simulink model "PF70mmDuctFanP"  (R2018b)
settings: Solver=ode4  StartTime=0.0  StopTime=10.0  RelTol=1e-3
libraries: simulink x1, vrlib x1
settings Model: Creator=sweat  LastModifiedBy=39926

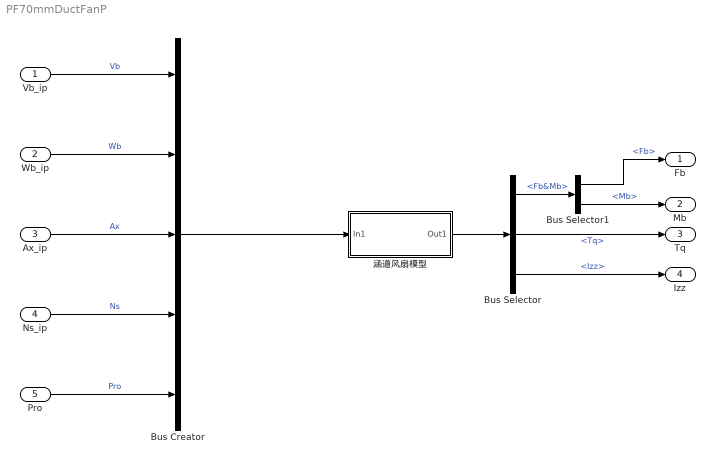
== system PF70mmDuctFanP ==
  Vb_ip : Inport  PortDimensions=3
  Wb_ip : Inport  Port=2  PortDimensions=3
  Ax_ip : Inport  Port=3  PortDimensions=3
  Ns_ip : Inport  Port=4  PortDimensions=1
  Pro : Inport  Port=5  PortDimensions=1
  Bus Selector : BusSelector  OutputSignals=Fb&Mb,Tq,Izz
  Bus Selector1 : BusSelector  OutputSignals=Fb,Mb
  Bus Creator : BusCreator  Inputs=5
  "涵道风扇模型 " : Subsystem  mask{Fratio=1.125, Mratio=0.975, Tqratio=0.4, Izz=0.00000309}
      mask prompts: Fratio "涵道风扇气动力修正系数"; Mratio "涵道风扇气动力矩修正系数"; Tqratio "涵道风扇扭矩修正系数"; Izz "涵道风扇转动惯量"
  Fb : Outport
  Mb : Outport  Port=2
  Tq : Outport  Port=3
  Izz : Outport  Port=4
  wires:
  Vb_ip/1 -> Bus Creator/1  "Vb"
  Wb_ip/1 -> Bus Creator/2  "Wb"
  Ax_ip/1 -> Bus Creator/3  "Ax"
  Ns_ip/1 -> Bus Creator/4  "Ns"
  Pro/1 -> Bus Creator/5  "Pro"
  Bus Creator/1 -> "涵道风扇模型 "/1(In1)
  "涵道风扇模型 "/1(Out1) -> Bus Selector/1
  Bus Selector/1 -> Bus Selector1/1  "<Fb&Mb>"
  Bus Selector1/1 -> Fb/1  "<Fb>"
  Bus Selector1/2 -> Mb/1  "<Mb>"
  Bus Selector/2 -> Tq/1  "<Tq>"
  Bus Selector/3 -> Izz/1  "<Izz>"

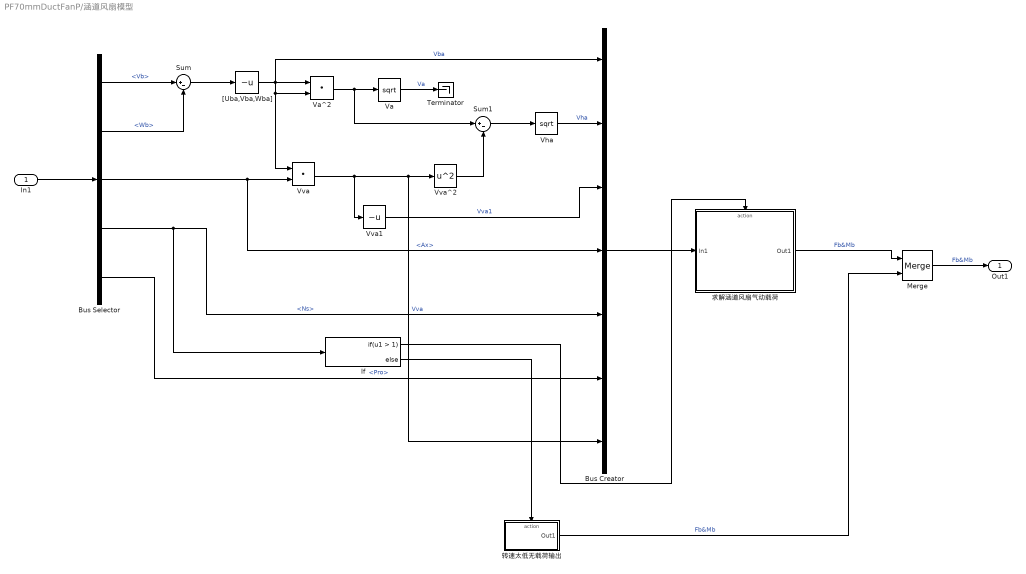
== system PF70mmDuctFanP/涵道风扇模型  ==
  In1 : Inport
  Bus Creator : BusCreator  Inputs=7
  Bus Selector : BusSelector  OutputSignals=Vb,Wb,Ax,Ns,Pro
  If : If  IfExpression=u1 > 1
  Merge : Merge
  Sum : Sum  Inputs=|+-
  Sum1 : Sum  Inputs=|+-
  Terminator : Terminator
  Va : Sqrt  SaturateOnIntegerOverflow=on
  Va^2 : DotProduct  InputSameDT=on  OutDataTypeStr=Inherit: Inherit via internal rule
  Vha : Sqrt  SaturateOnIntegerOverflow=on
  Vva : DotProduct  InputSameDT=on  OutDataTypeStr=Inherit: Inherit via internal rule
  Vva1 : UnaryMinus
  Vva^2 : Math  Operator=square  SaturateOnIntegerOverflow=on
  "[Uba,Vba,Wba]" : UnaryMinus
  求解涵道风扇气动载荷 : Subsystem  TreatAsAtomicUnit=on
  转速太低无载荷输出 : Subsystem  TreatAsAtomicUnit=on
  Out1 : Outport
  wires:
  Bus Selector/1 -> Sum/1  "<Vb>"
  In1/1 -> Bus Selector/1
  Bus Selector/2 -> Sum/2  "<Wb>"
  Sum/1 -> "[Uba,Vba,Wba]"/1
  "[Uba,Vba,Wba]"/1 -> Bus Creator/1, Vva/1, Va^2/2, Va^2/1  "Vba"
  Bus Selector/3 -> Bus Creator/4, Vva/2  "<Ax>"
  Va^2/1 -> Sum1/1, Va/1
  Vva/1 -> Bus Creator/7, Vva^2/1, Vva1/1  "Vva"
  Vva^2/1 -> Sum1/2
  Sum1/1 -> Vha/1
  Vha/1 -> Bus Creator/2  "Vha"
  Vva1/1 -> Bus Creator/3  "Vva1"
  Bus Selector/4 -> Bus Creator/5, If/1  "<Ns>"
  If/1 -> 求解涵道风扇气动载荷/Action
  If/2 -> 转速太低无载荷输出/Action
  Bus Selector/5 -> Bus Creator/6  "<Pro>"
  Bus Creator/1 -> 求解涵道风扇气动载荷/1(In1)
  求解涵道风扇气动载荷/1(Out1) -> Merge/1  "Fb&Mb"
  转速太低无载荷输出/1(Out1) -> Merge/2  "Fb&Mb"
  Va/1 -> Terminator/1  "Va"
  Merge/1 -> Out1/1  "Fb&Mb"

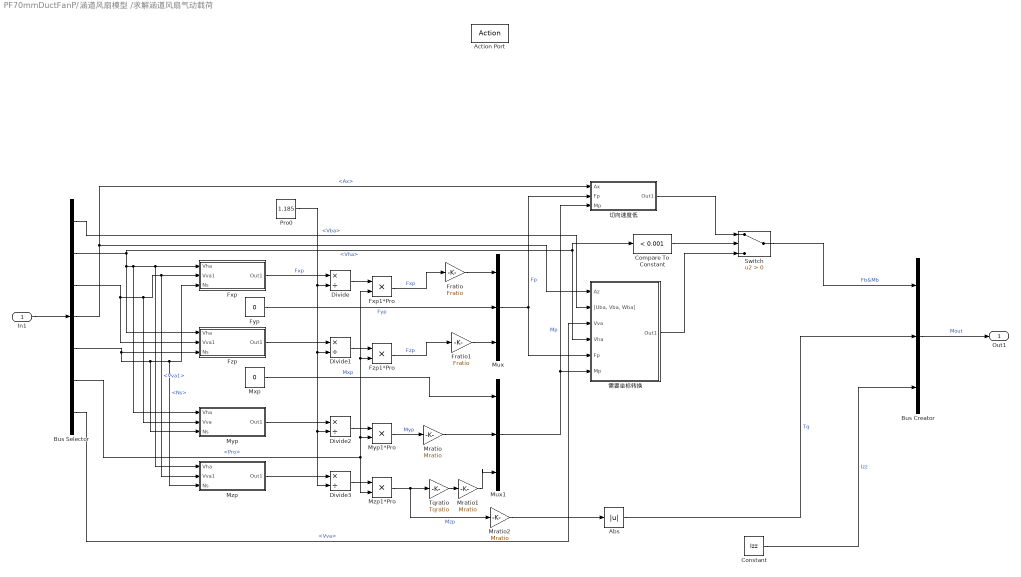
== system PF70mmDuctFanP/涵道风扇模型 /求解涵道风扇气动载荷 ==
  In1 : Inport
  Action Port : ActionPort  ActionType=then
  Abs : Abs
  Bus Creator : BusCreator  Inputs=3
  Bus Selector : BusSelector  OutputSignals=Vba,Vha,Vva1,Ax,Ns,Pro,Vva
  Compare To Constant : simulink/Logic and Bit Operations/Compare To Constant  relop=<  const=0.001  OutDataTypeStr=boolean
  Constant : Constant  Value=Izz
  Divide{,1..3} (4 alike) : Product  Inputs=*/
  Fratio : Gain  Gain=Fratio
  Fratio1 : Gain  Gain=Fratio
  Fxp : Subsystem
  Fxp1*Pro : Product
  Fyp : Constant  Value=0
  Fzp : Subsystem
  Fzp1*Pro : Product
  Mratio : Gain  Gain=Mratio
  Mratio1 : Gain  Gain=Mratio
  Mratio2 : Gain  Gain=Mratio
  Mux : Mux  Inputs=3
  Mux1 : Mux  Inputs=3
  Mxp : Constant  Value=0
  Myp : Subsystem
  Myp1*Pro : Product
  Mzp : Subsystem
  Mzp1*Pro : Product
  Pro0 : Constant  Value=1.185
  Switch : Switch  Criteria=u2 > Threshold
  Tqratio : Gain  Gain=Tqratio
  切向速度低 : Subsystem
  需要坐标转换 : Subsystem
  Out1 : Outport
  wires:
  In1/1 -> Bus Selector/1
  Bus Selector/2 -> Fzp/1(Vha), Myp/1(Vha), Mzp/1(Vha), Fxp/1(Vha), 需要坐标转换/4(Vha), Compare To Constant/1  "<Vha>"
  Bus Selector/3 -> Myp/2(Vva), Mzp/2(Vva1), Fxp/2(Vva1), Fzp/2(Vva1)  "<Vva1>"
  Bus Selector/5 -> Fzp/3(Ns), Myp/3(Ns), Mzp/3(Ns), Fxp/3(Ns)  "<Ns>"
  Fyp/1 -> Mux/2  "Fyp"
  Fxp/1(Out1) -> Divide/1  "Fxp"
  Fzp/1(Out1) -> Divide1/1
  Myp/1(Out1) -> Divide2/1
  Mzp/1(Out1) -> Divide3/1
  Pro0/1 -> Divide3/2, Divide2/2, Divide1/2, Divide/2
  Divide/1 -> Fxp1*Pro/1
  Fxp1*Pro/1 -> Fratio/1  "Fxp"
  Divide1/1 -> Fzp1*Pro/1
  Fzp1*Pro/1 -> Fratio1/1  "Fzp"
  Bus Selector/6 -> Mzp1*Pro/2, Myp1*Pro/2, Fzp1*Pro/2, Fxp1*Pro/2  "<Pro>"
  Divide2/1 -> Myp1*Pro/1
  Myp1*Pro/1 -> Mratio/1  "Myp"
  Divide3/1 -> Mzp1*Pro/1
  Bus Selector/4 -> 需要坐标转换/1(Az), 切向速度低/1(Ax)  "<Ax>"
  Mux/1 -> 需要坐标转换/5(Fp), 切向速度低/2(Fp)  "Fp"
  Mux1/1 -> 需要坐标转换/6(Mp), 切向速度低/3(Mp)  "Mp"
  Bus Selector/1 -> 需要坐标转换/2("[Uba, Vba, Wba]")  "<Vba>"
  Bus Selector/7 -> 需要坐标转换/3(Vva)  "<Vva>"
  Compare To Constant/1 -> Switch/2
  需要坐标转换/1(Out1) -> Switch/3
  Abs/1 -> Bus Creator/2  "Tq"
  Mzp1*Pro/1 -> Mratio2/1, Tqratio/1  "Mzp"
  Fratio/1 -> Mux/1
  Fratio1/1 -> Mux/3
  Tqratio/1 -> Mratio1/1
  Mratio/1 -> Mux1/2
  Mratio1/1 -> Mux1/3
  Mratio2/1 -> Abs/1
  Constant/1 -> Bus Creator/3  "Izz"
  Switch/1 -> Bus Creator/1  "Fb&Mb"
  Bus Creator/1 -> Out1/1  "Mout"
  切向速度低/1(Out1) -> Switch/1
  Mxp/1 -> Mux1/1  "Mxp"

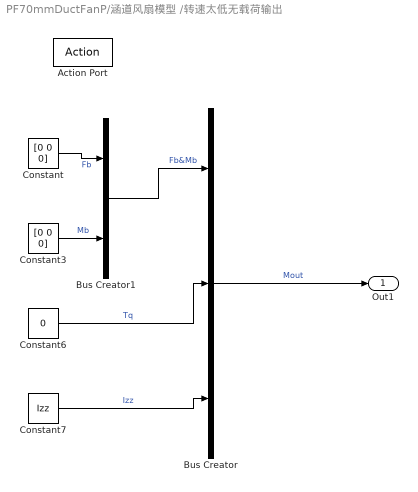
== system PF70mmDuctFanP/涵道风扇模型 /转速太低无载荷输出 ==
  Action Port : ActionPort  ActionType=else
  Bus Creator : BusCreator  Inputs=3
  Bus Creator1 : BusCreator  Inputs=2
  Constant : Constant  Value=[0 0 0]
  Constant3 : Constant  Value=[0 0 0]
  Constant6 : Constant  Value=0
  Constant7 : Constant  Value=Izz
  Out1 : Outport
  wires:
  Constant6/1 -> Bus Creator/2  "Tq"
  Constant7/1 -> Bus Creator/3  "Izz"
  Bus Creator/1 -> Out1/1  "Mout"
  Constant/1 -> Bus Creator1/1  "Fb"
  Constant3/1 -> Bus Creator1/2  "Mb"
  Bus Creator1/1 -> Bus Creator/1  "Fb&Mb"

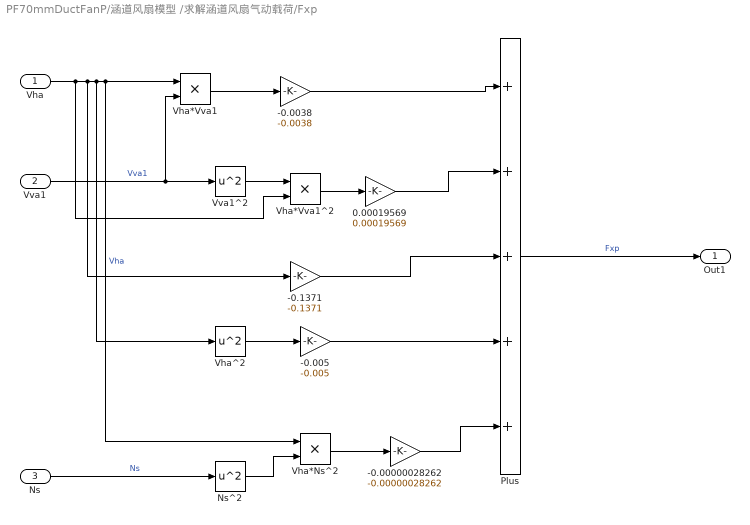
== system PF70mmDuctFanP/涵道风扇模型 /求解涵道风扇气动载荷/Fxp ==
  Vha : Inport
  Vva1 : Inport  Port=2
  Ns : Inport  Port=3
  -0.00000028262 : Gain  Gain=-0.00000028262
  -0.0038 : Gain  Gain=-0.0038
  -0.005 : Gain  Gain=-0.005
  -0.1371 : Gain  Gain=-0.1371
  0.00019569 : Gain  Gain=0.00019569
  Ns^2 : Math  Operator=square  SaturateOnIntegerOverflow=on
  Plus : Sum  Inputs=+++++
  Vha*Ns^2 : Product
  Vha*Vva1 : Product
  Vha*Vva1^2 : Product
  Vha^2 : Math  Operator=square  SaturateOnIntegerOverflow=on
  Vva1^2 : Math  Operator=square  SaturateOnIntegerOverflow=on
  Out1 : Outport
  wires:
  Vha/1 -> Vha*Vva1^2/2, -0.1371/1, Vha^2/1, Vha*Ns^2/1, Vha*Vva1/1  "Vha"
  Vva1/1 -> Vva1^2/1, Vha*Vva1/2  "Vva1"
  Vha*Vva1/1 -> -0.0038/1
  -0.0038/1 -> Plus/1
  Ns/1 -> Ns^2/1  "Ns"
  Vva1^2/1 -> Vha*Vva1^2/1
  Vha*Vva1^2/1 -> 0.00019569/1
  0.00019569/1 -> Plus/2
  -0.1371/1 -> Plus/3
  Vha^2/1 -> -0.005/1
  -0.005/1 -> Plus/4
  Ns^2/1 -> Vha*Ns^2/2
  Vha*Ns^2/1 -> -0.00000028262/1
  -0.00000028262/1 -> Plus/5
  Plus/1 -> Out1/1  "Fxp"

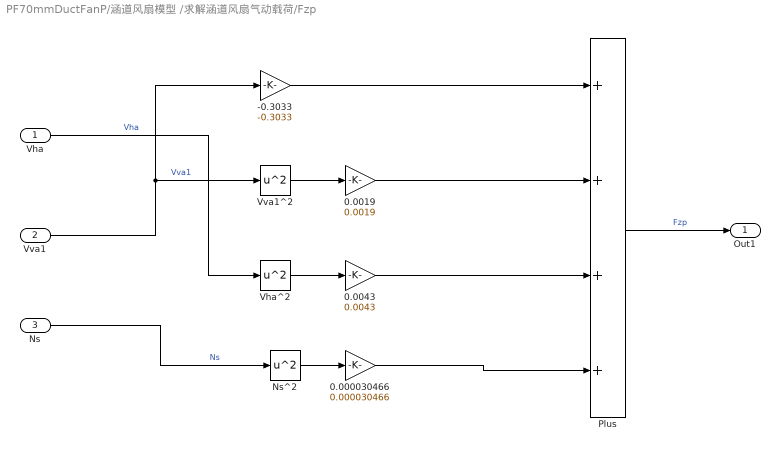
== system PF70mmDuctFanP/涵道风扇模型 /求解涵道风扇气动载荷/Fzp ==
  Vha : Inport
  Vva1 : Inport  Port=2
  Ns : Inport  Port=3
  -0.3033 : Gain  Gain=-0.3033
  0.000030466 : Gain  Gain=0.000030466
  0.0019 : Gain  Gain=0.0019
  0.0043 : Gain  Gain=0.0043
  Ns^2 : Math  Operator=square  SaturateOnIntegerOverflow=on
  Plus : Sum  Inputs=++++
  Vha^2 : Math  Operator=square  SaturateOnIntegerOverflow=on
  Vva1^2 : Math  Operator=square  SaturateOnIntegerOverflow=on
  Out1 : Outport
  wires:
  Vha/1 -> Vha^2/1  "Vha"
  Vva1/1 -> -0.3033/1, Vva1^2/1  "Vva1"
  Ns/1 -> Ns^2/1  "Ns"
  -0.3033/1 -> Plus/1
  Vva1^2/1 -> 0.0019/1
  0.0019/1 -> Plus/2
  Vha^2/1 -> 0.0043/1
  0.0043/1 -> Plus/3
  Ns^2/1 -> 0.000030466/1
  0.000030466/1 -> Plus/4
  Plus/1 -> Out1/1  "Fzp"

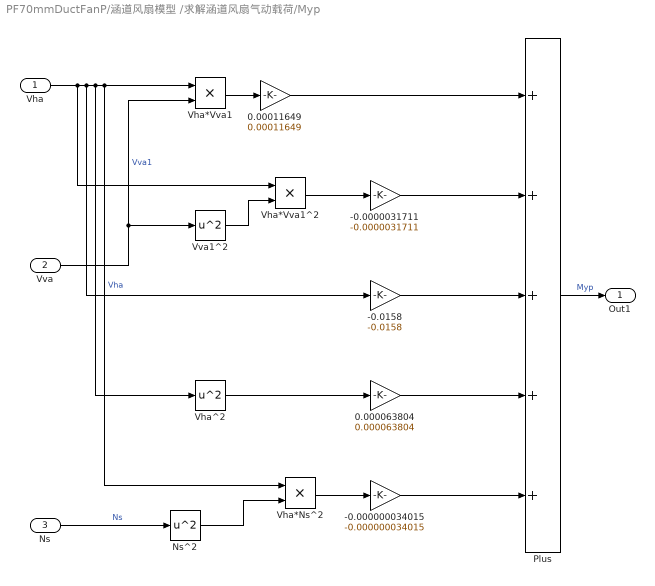
== system PF70mmDuctFanP/涵道风扇模型 /求解涵道风扇气动载荷/Myp ==
  Vha : Inport
  Vva : Inport  Port=2
  Ns : Inport  Port=3
  -0.000000034015 : Gain  Gain=-0.000000034015
  -0.0000031711 : Gain  Gain=-0.0000031711
  -0.0158 : Gain  Gain=-0.0158
  0.000063804 : Gain  Gain=0.000063804
  0.00011649 : Gain  Gain=0.00011649
  Ns^2 : Math  Operator=square  SaturateOnIntegerOverflow=on
  Plus : Sum  Inputs=+++++
  Vha*Ns^2 : Product
  Vha*Vva1 : Product
  Vha*Vva1^2 : Product
  Vha^2 : Math  Operator=square  SaturateOnIntegerOverflow=on
  Vva1^2 : Math  Operator=square  SaturateOnIntegerOverflow=on
  Out1 : Outport
  wires:
  Vha/1 -> Vha*Vva1^2/1, -0.0158/1, Vha^2/1, Vha*Ns^2/1, Vha*Vva1/1  "Vha"
  Vva/1 -> Vha*Vva1/2, Vva1^2/1  "Vva1"
  Ns/1 -> Ns^2/1  "Ns"
  Plus/1 -> Out1/1  "Myp"
  Vha*Vva1/1 -> 0.00011649/1
  0.00011649/1 -> Plus/1
  Vha*Vva1^2/1 -> -0.0000031711/1
  -0.0000031711/1 -> Plus/2
  Vva1^2/1 -> Vha*Vva1^2/2
  -0.0158/1 -> Plus/3
  Vha^2/1 -> 0.000063804/1
  0.000063804/1 -> Plus/4
  -0.000000034015/1 -> Plus/5
  Vha*Ns^2/1 -> -0.000000034015/1
  Ns^2/1 -> Vha*Ns^2/2

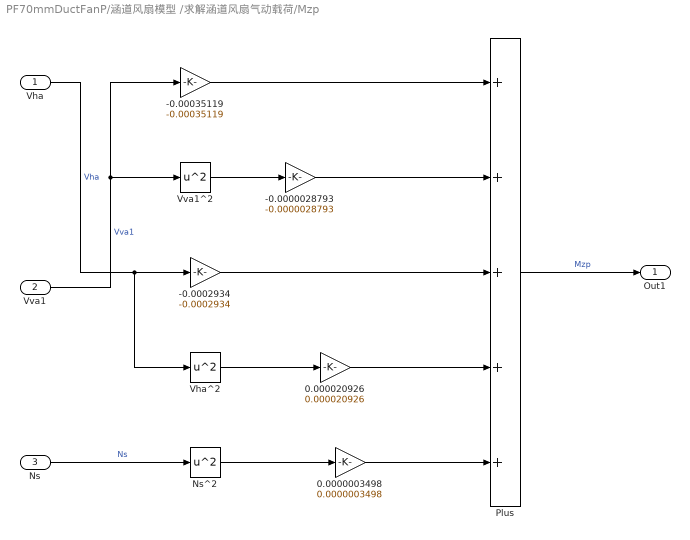
== system PF70mmDuctFanP/涵道风扇模型 /求解涵道风扇气动载荷/Mzp ==
  Vha : Inport
  Vva1 : Inport  Port=2
  Ns : Inport  Port=3
  -0.0000028793 : Gain  Gain=-0.0000028793
  -0.0002934 : Gain  Gain=-0.0002934
  -0.00035119 : Gain  Gain=-0.00035119
  "0.0000003498 " : Gain  Gain=0.0000003498
  0.000020926 : Gain  Gain=0.000020926
  Ns^2 : Math  Operator=square  SaturateOnIntegerOverflow=on
  Plus : Sum  Inputs=+++++
  Vha^2 : Math  Operator=square  SaturateOnIntegerOverflow=on
  Vva1^2 : Math  Operator=square  SaturateOnIntegerOverflow=on
  Out1 : Outport
  wires:
  Plus/1 -> Out1/1  "Mzp"
  Vha/1 -> Vha^2/1, -0.0002934/1  "Vha"
  Vva1/1 -> Vva1^2/1, -0.00035119/1  "Vva1"
  Ns/1 -> Ns^2/1  "Ns"
  -0.00035119/1 -> Plus/1
  -0.0000028793/1 -> Plus/2
  Vva1^2/1 -> -0.0000028793/1
  -0.0002934/1 -> Plus/3
  0.000020926/1 -> Plus/4
  Vha^2/1 -> 0.000020926/1
  "0.0000003498 "/1 -> Plus/5
  Ns^2/1 -> "0.0000003498 "/1

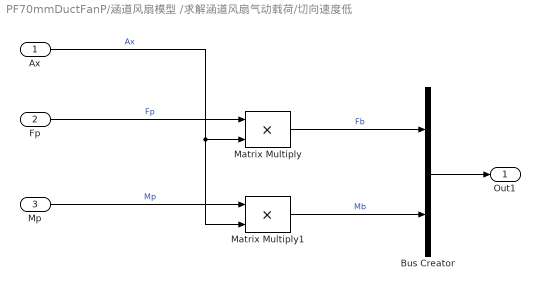
== system PF70mmDuctFanP/涵道风扇模型 /求解涵道风扇气动载荷/切向速度低 ==
  Ax : Inport
  Fp : Inport  Port=2
  Mp : Inport  Port=3
  Bus Creator : BusCreator  Inputs=2
  Matrix Multiply : Product
  Matrix Multiply1 : Product
  Out1 : Outport
  wires:
  Ax/1 -> Matrix Multiply1/2, Matrix Multiply/2  "Ax"
  Fp/1 -> Matrix Multiply/1  "Fp"
  Mp/1 -> Matrix Multiply1/1  "Mp"
  Bus Creator/1 -> Out1/1
  Matrix Multiply/1 -> Bus Creator/1  "Fb"
  Matrix Multiply1/1 -> Bus Creator/2  "Mb"

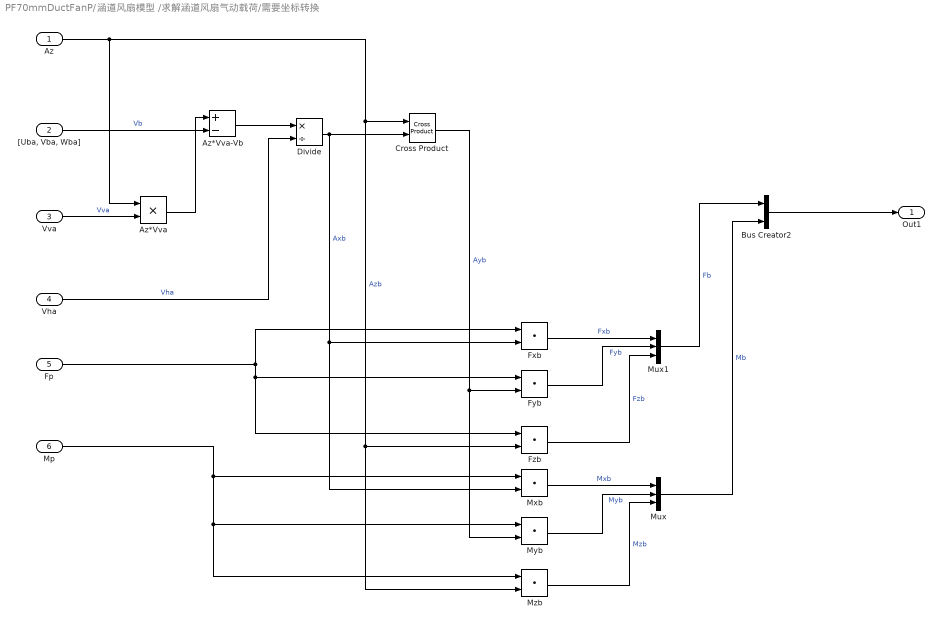
== system PF70mmDuctFanP/涵道风扇模型 /求解涵道风扇气动载荷/需要坐标转换 ==
  Az : Inport
  "[Uba, Vba, Wba]" : Inport  Port=2
  Vva : Inport  Port=3
  Vha : Inport  Port=4
  Fp : Inport  Port=5
  Mp : Inport  Port=6
  Az*Vva : Product
  Az*Vva-Vb : Sum  Inputs=+-
  Bus Creator2 : BusCreator  Inputs=2
  Cross Product : vrlib/Utilities/Cross Product
      settings: SourceProductBaseCode=VR
  Divide : Product  Inputs=*/
  Fxb : DotProduct  InputSameDT=on  OutDataTypeStr=Inherit: Inherit via internal rule
  Fyb : DotProduct  InputSameDT=on  OutDataTypeStr=Inherit: Inherit via internal rule
  Fzb : DotProduct  InputSameDT=on  OutDataTypeStr=Inherit: Inherit via internal rule
  Mux : Mux  Inputs=3
  Mux1 : Mux  Inputs=3
  Mxb : DotProduct  InputSameDT=on  OutDataTypeStr=Inherit: Inherit via internal rule
  Myb : DotProduct  InputSameDT=on  OutDataTypeStr=Inherit: Inherit via internal rule
  Mzb : DotProduct  InputSameDT=on  OutDataTypeStr=Inherit: Inherit via internal rule
  Out1 : Outport
  wires:
  Vva/1 -> Az*Vva/2  "Vva"
  Az/1 -> Cross Product/1, Fzb/2, Mzb/2, Az*Vva/1  "Azb"
  Az*Vva/1 -> Az*Vva-Vb/1
  "[Uba, Vba, Wba]"/1 -> Az*Vva-Vb/2  "Vb"
  Az*Vva-Vb/1 -> Divide/1
  Vha/1 -> Divide/2  "Vha"
  Divide/1 -> Cross Product/2, Mxb/2, Fxb/2  "Axb"
  Cross Product/1 -> Myb/2, Fyb/2  "Ayb"
  Fp/1 -> Fzb/1, Fyb/1, Fxb/1
  Mp/1 -> Mzb/1, Myb/1, Mxb/1
  Fxb/1 -> Mux1/1  "Fxb"
  Fyb/1 -> Mux1/2  "Fyb"
  Fzb/1 -> Mux1/3  "Fzb"
  Mxb/1 -> Mux/1  "Mxb"
  Myb/1 -> Mux/2  "Myb"
  Mzb/1 -> Mux/3  "Mzb"
  Mux1/1 -> Bus Creator2/1  "Fb"
  Mux/1 -> Bus Creator2/2  "Mb"
  Bus Creator2/1 -> Out1/1
